simulink model "AeroDynamicLevitationInputGU_2020b"  (R2023b)
settings: Solver=FixedStepAuto  StartTime=0.0  StopTime=inf  RelTol=1e-3
undefined symbols (not defined in the file): National_Instruments, PCIe
libraries: sldrtlib x2
settings Model: Creator=maincurvati  LastModifiedBy=fluky
settings SolverCC: AlgebraicLoopSolver=TrustRegion
settings DataIOCC: ReturnWorkspaceOutputs=off
settings DebuggingCC: UnconnectedInputMsg=warning  UnconnectedOutputMsg=warning  UnconnectedLineMsg=warning  ArithmeticOperatorsInVariantConditions=warning
settings HardwareCC: ProdBitPerLong=64  ProdHWDeviceType=Intel->x86-64 (Linux 64)
settings ModelReferenceCC: EnableRefExpFcnMdlSchedulingChecks=on
settings SFSimCC: SimUseLocalCustomCode=off  CustomCodeUndefinedFunction=UseInterfaceOnly
settings RTWCC: Description=Simulink Desktop Real-Time  SystemTargetFile=sldrt.tlc  TemplateMakefile=sldrt.tmf  RTWUseLocalCustomCode=off  RTWCompilerOptimization=on  DLArmComputeVersion=19.05
settings CodeAppCC: MaxIdLength=95  StateflowObjectComments=on
settings SimulinkDesktopRealTimeCC: TargetLibSuffix=_sldrt.a  TargetPreCompLibLocation=C:\Program Files\MATLAB\R2023b\toolbox\sldrt\lib\win64

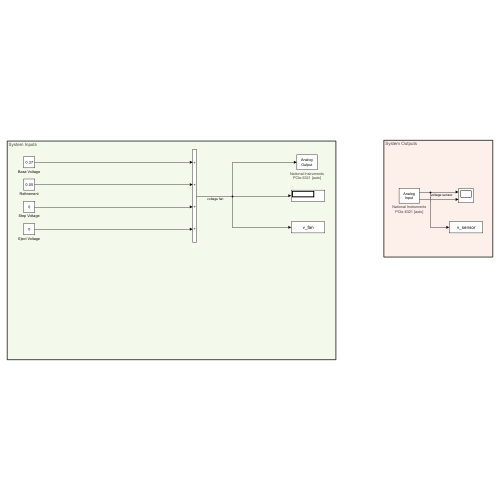
[thumbnail: Simulink's stored preview of the top-level diagram]
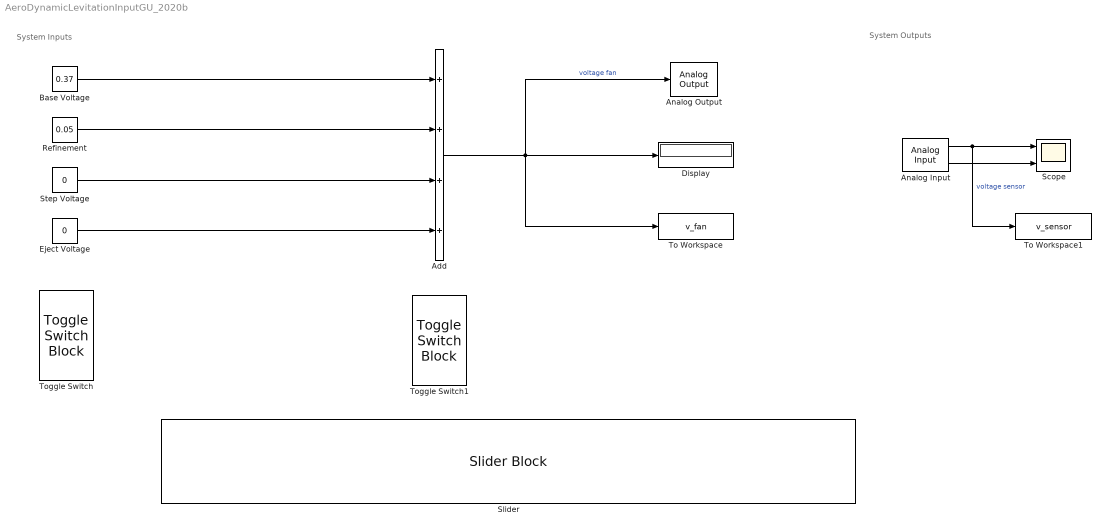
== system AeroDynamicLevitationInputGU_2020b ==
  note: System Outputs
  note: System Inputs
  Add : Sum  Inputs=++++
  Analog Input : sldrtlib/Analog Input  SampleTime=0.002  MaxMissedTicks=1000  ShowMissedTicks=on  YieldWhenWaiting=off  DrvName=National_Instruments/PCIe-6321  DrvAddress=4294967295  DrvOptions=[0 0 0 0 0 0 0]  Channels=1  RangeMode=1  VoltRange=1  DataType=1
      settings: AttributesFormatString=National Instruments\nPCIe-6321 [auto]
  Analog Output : sldrtlib/Analog Output  SampleTime=2e-3  MaxMissedTicks=1000  ShowMissedTicks=off  YieldWhenWaiting=off  DrvName=National_Instruments/PCIe-6321  DrvAddress=4294967295  DrvOptions=[0 0 0 0 0 0 0]  Channels=1  RangeMode=1  VoltRange=1  InitialValue=0  FinalValue=0
      settings: AttributesFormatString=National Instruments\nPCIe-6321 [auto]
  Base Voltage : Constant  Value=0.37
  Display : Display
  Eject Voltage : Constant  Value=0
  Refinement : Constant  Value=0.05
  Scope : Scope  NumInputPorts=2
  Slider : SliderBlock  ScaleMax=0.1
  Step Voltage : Constant  Value=0
  To Workspace : ToWorkspace  VariableName=v_fan  SaveFormat=Timeseries  SampleTime=2e-3
  To Workspace1 : ToWorkspace  VariableName=v_sensor  SaveFormat=Timeseries  SampleTime=2e-3
  Toggle Switch : ToggleSwitchBlock
      settings: Values={{'Off', 'On'}, [0 0.02]}
  Toggle Switch1 : ToggleSwitchBlock
      settings: Values={{'Off', 'On'}, [0 1]}
  wires:
  Add/1 -> Analog Output/1, To Workspace/1, Display/1  "voltage fan"
  Step Voltage/1 -> Add/3
  Base Voltage/1 -> Add/1
  Analog Input/1 -> Scope/1, To Workspace1/1  "voltage sensor"
  Analog Input/2 -> Scope/2
  Eject Voltage/1 -> Add/4
  Refinement/1 -> Add/2
